simulink model "Part4_2_1"  (R2021a)
settings: Solver=VariableStepAuto  StartTime=0.0  StopTime=2000  RelTol=1e-3
undefined symbols (not defined in the file or in its folder): quant
settings Model: Creator=theod  LastModifiedBy=theod

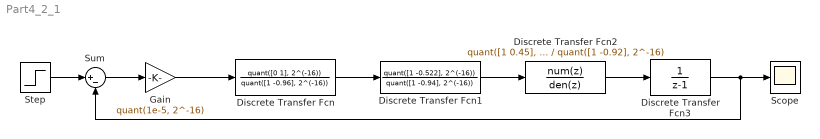
== system Part4_2_1 ==
  Discrete Transfer Fcn : DiscreteTransferFcn  Numerator=quant([0 1], 2^(-16))  Denominator=quant([1 -0.96], 2^(-16))
  Discrete Transfer Fcn1 : DiscreteTransferFcn  Numerator=quant([1 -0.522], 2^(-16))  Denominator=quant([1 -0.94], 2^(-16))
  Discrete Transfer Fcn2 : DiscreteTransferFcn  Numerator=quant([1 0.45], 2^(-16))  Denominator=quant([1 -0.92], 2^-16)
  Discrete Transfer Fcn3 : DiscreteTransferFcn  Denominator=[1 -1]
  Gain : Gain  Gain=quant(1e-5, 2^-16)
  Scope : Scope
  Step : Step  SampleTime=0.1
  Sum : Sum  Inputs=|+-
  wires:
  Discrete Transfer Fcn/1 -> Discrete Transfer Fcn1/1
  Discrete Transfer Fcn1/1 -> Discrete Transfer Fcn2/1
  Discrete Transfer Fcn2/1 -> Discrete Transfer Fcn3/1
  Gain/1 -> Discrete Transfer Fcn/1
  Step/1 -> Sum/1
  Sum/1 -> Gain/1
  Discrete Transfer Fcn3/1 -> Sum/2, Scope/1
